simulink model "test_single_phase_contactor"  (R2017b)
settings: Solver=VariableStepAuto  StartTime=0.0  StopTime=10.0  RelTol=1e-3
undefined symbols (not defined in the file): S2
libraries: powerlib x3, typhoonHILlib x1
settings Model: Creator=Marcos  LastModifiedBy=Marcos

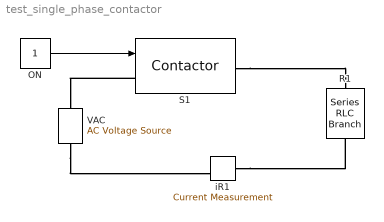
== system test_single_phase_contactor ==
  ON : Constant
  R1 : powerlib/Elements/Series RLC Branch  LConnTagsString=__new0  RConnTagsString=__new0  BranchType=R  Resistance=10  Inductance=1e-3  SetiL0=off  InitialCurrent=0  Capacitance=1e-6  Setx0=off  InitialVoltage=0  Measurements=None
  S1 : typhoonHILlib/Contactor  ContType=Single Pole Single Throw  init_state=Off / S2  s1_logic=Active-high  di_1=1  tr1_delay=0  tr2_delay=0  r_on=0.001  v_f=0  r_s=1e4  c_s=inf  s0=0  toggle_init=on  old_pat=typhoonPatterns/SPST Contactor  old_size=100,55  model_loaded=off
      settings: SourceProductName=Typhoon HIL
  VAC : powerlib/Electrical Sources/AC Voltage Source  Amplitude=311.127  Phase=0  Frequency=50  SampleTime=0  Measurements=None  BusType=swing  Pref=10e3  Qref=0  Qmin=-inf  Qmax=+inf
  iR1 : powerlib/Measurements/Current Measurement  PhasorSimulation=off  OutputType=Complex  PSBequivalent=0
  wires:
  ON/1 -> S1/1
  connections:
  S1/RConn1 -- R1/LConn1
  VAC/LConn1 -- iR1/RConn1
  iR1/LConn1 -- R1/RConn1
  S1/LConn1 -- VAC/RConn1
